simulink model "ASM"  (R2019a)
settings: Solver=VariableStepAuto  StartTime=0.0  StopTime=10.0  RelTol=1e-3
libraries: powerlib x9, simulink x2
settings Model: Creator=amank  LastModifiedBy=amank

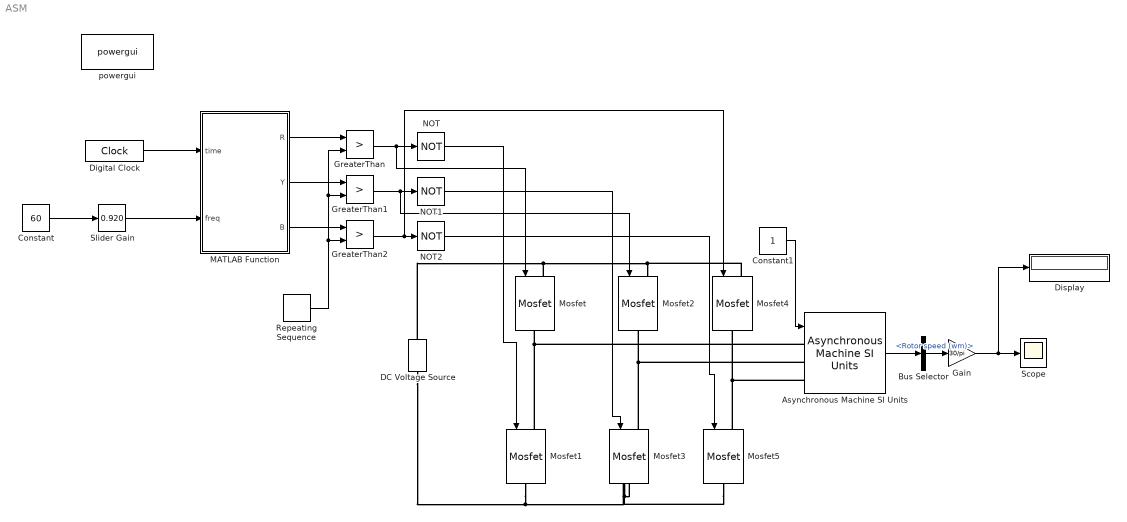
== system ASM ==
  Asynchronous Machine SI Units : powerlib/Machines/Asynchronous Machine SI Units  RotorType=Squirrel-cage  PresetModel="07:  200 HP 460 V 60Hz 1785 RPM"  MechanicalLoad=Torque Tm  ShowDetailedParameters=on  ReferenceFrame=Rotor  Units=SI  MeasurementBus=off  NominalParameters=[1.492e+05 460 60]  Stator=[0.01818 0.00019]  Rotor=[0.009956 0.00019]  Cage1=[0.4155 0.002066]  Cage2=[0.4168 0.0003495]  Lm=0.009415  Mechanical=[2.6 0.04789 2]  PolePairs=2  InitialConditions=[0 0 0 0 0 0 0 0]  SimulateSaturation=off  Saturation=[14.03593122, 27.81365428, 53.79336849, 72.68890987, 97.98006896, 148.6815601, 215.7428561, 302.9841135, 428.7778367 ; 230, 322, 414, 460, 506, 552, 598, 644, 690]  LoadFlowParameters=1492000  TsPowergui=0  TsBlock=-1  IterativeModel=Trapezoidal non iterative  IterativeDiscreteModel=Trapezoidal non iterative  Pmec=1.492e+006
      settings: SourceProductName=Simscape Electrical
  Bus Selector : BusSelector  OutputSignals=Mechanical.Rotor speed (wm)
  Constant : Constant  Value=60
  Constant1 : Constant
  DC Voltage Source : powerlib/Electrical Sources/DC Voltage Source  Amplitude=500  Measurements=None
      settings: SourceProductName=Simscape Electrical
  Digital Clock : DigitalClock  SampleTime=1e-5
  Display : Display
  Gain : Gain  Gain=30/pi
  GreaterThan : RelationalOperator  Operator=>  OutDataTypeStr=boolean  RndMeth=Simplest
  GreaterThan1 : RelationalOperator  Operator=>  OutDataTypeStr=boolean  RndMeth=Simplest
  GreaterThan2 : RelationalOperator  Operator=>  OutDataTypeStr=boolean  RndMeth=Simplest
  MATLAB Function : MATLAB Function  TreatAsAtomicUnit=on
  Mosfet{,1..5} (6 alike) : powerlib/Power Electronics/Mosfet  Ron=0.1  Lon=0  Rd=0.01  Vfd=0  IC=0  Rs=1e5  Cs=inf  Measurements=off
      settings: SourceProductName=Simscape Electrical
  NOT : Logic  Operator=NOT  IconShape=distinctive  AllPortsSameDT=off  OutDataTypeStr=boolean
  NOT1 : Logic  Operator=NOT  IconShape=distinctive  AllPortsSameDT=off  OutDataTypeStr=boolean
  NOT2 : Logic  Operator=NOT  IconShape=distinctive  AllPortsSameDT=off  OutDataTypeStr=boolean
  Repeating Sequence : simulink/Sources/Repeating Sequence  rep_seq_t=[0 .25 .5 .75 1]*1/5000  rep_seq_y=[0 1 0 -1 0]
  Scope : Scope
  Slider Gain : simulink/Math Operations/Slider Gain  gain=0.920  low=0  high=1
  powergui : powerlib/powergui  Priority=1  SimulationMode=Discrete  SampleTime=1e-5  frequency=60  Iterations=50  frequencyindice=60  Pbase=100e6  ErrMax=1e-4  UnitsV=kV  UnitsW=MW  buscounter=0  FunctionMessages=off  echomessages=off  EnableUseOfTLC=off  CurrentSourceSwitches=off  DisableSnubberDevices=off  DisableRonSwitches=off  DisableVfSwitches=off  DisplayEquations=off  AutomaticDiscreteSolvers=off  SolverType=Tustin/Backward Euler (TBE)  Interpol=off  ExternalGateDelay=off  methode=off  Ts=100  x0status=blocks  SPID=on  SwTol=0  HookPort=off  NonlinearTolerance=0  nMaxIteration=15  ContinueOnMaxIteration=off  RestoreLinks=warning  ResistiveCurrentMeasurement=off  Frange=[0:2:500]  Ylog=off  Xlog=on  ShowGrid=off  save=off  variable=ZData  structure=0  ZoomFFT=off  StartTime=0.0  cycles=1  DisplayStyle=1  fundamental=60  FreqAxis=off  MaxFrequency=1000  frequencyindicesteady=1  RmsSteady=1  display=off
      settings: SourceProductName=Simscape Electrical
  wires:
  Constant/1 -> Slider Gain/1
  Slider Gain/1 -> MATLAB Function/2(freq)
  Digital Clock/1 -> MATLAB Function/1(time)
  MATLAB Function/1(R) -> GreaterThan/1
  MATLAB Function/2(Y) -> GreaterThan1/1
  MATLAB Function/3(B) -> GreaterThan2/1
  Repeating Sequence/1 -> GreaterThan2/2, GreaterThan1/2, GreaterThan/2
  GreaterThan/1 -> Mosfet/1, NOT/1
  GreaterThan1/1 -> Mosfet2/1, NOT1/1
  GreaterThan2/1 -> Mosfet4/1, NOT2/1
  NOT/1 -> Mosfet1/1
  NOT1/1 -> Mosfet3/1
  NOT2/1 -> Mosfet5/1
  Constant1/1 -> Asynchronous Machine SI Units/1
  Asynchronous Machine SI Units/1 -> Bus Selector/1
  Bus Selector/1 -> Gain/1  "<Rotor speed (wm)>"
  Gain/1 -> Display/1, Scope/1
  connections:
  Mosfet1/LConn1 -- Asynchronous Machine SI Units/LConn1 -- Mosfet/RConn1
  Mosfet3/LConn1 -- Asynchronous Machine SI Units/LConn2 -- Mosfet2/RConn1
  Mosfet5/LConn1 -- Asynchronous Machine SI Units/LConn3 -- Mosfet4/RConn1
  Mosfet/LConn1 -- Mosfet4/LConn1 -- Mosfet2/LConn1 -- DC Voltage Source/RConn1
  Mosfet1/RConn1 -- Mosfet5/RConn1 -- Mosfet3/RConn1 -- DC Voltage Source/LConn1

== matlab function ASM/MATLAB Function ==
  data: time input; R output; freq input; Y output; B output
function [R,Y,B] = fcn(time,freq)
omega=2*pi*freq;
R=sin(omega*time)*freq/60;
B=sin(omega*time+120*pi/180)*freq/60;
Y=sin(omega*time+240*pi/180)*freq/60;
